simulink model "buck_soft_start_logic"  (R2024b)
settings: Solver=ode4  StartTime=0.0  StopTime=0.018  FixedStep=5e-7  RelTol=1e-3
undefined symbols (not defined in the file): DiscIntNeverNeededParam
libraries: simulink x1
settings Model: Creator=ww  LastModifiedBy=ww

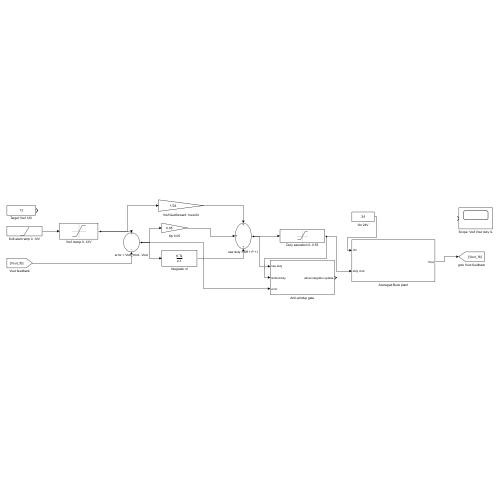
[thumbnail: Simulink's stored preview of the top-level diagram]
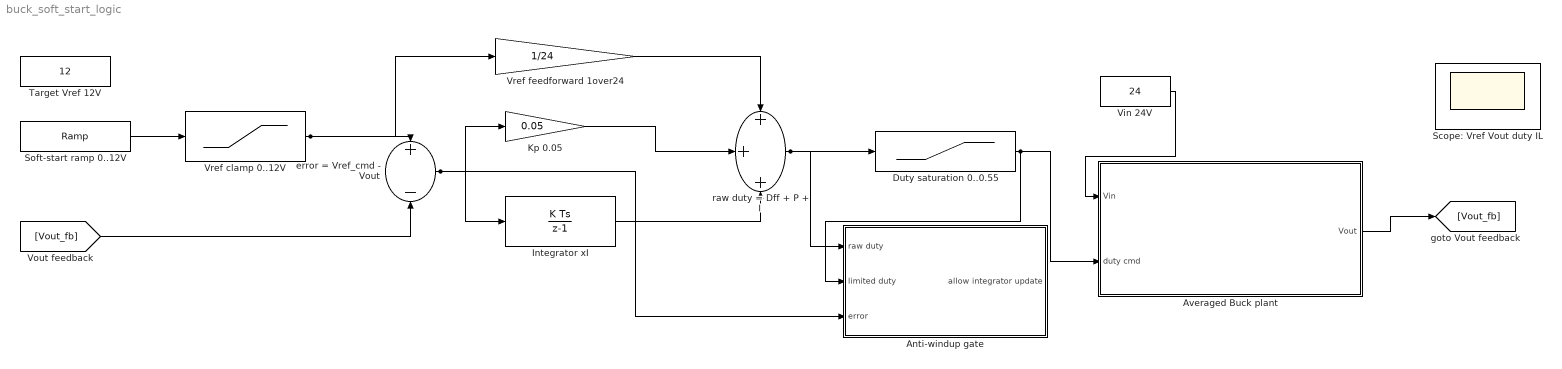
== system buck_soft_start_logic ==
  Anti-windup gate : Subsystem
  Averaged Buck plant : Subsystem
  Duty saturation 0..0.55 : Saturate  UpperLimit=0.55  LowerLimit=0
  Integrator xI : DiscreteIntegrator  gainval=200  SampleTime=5e-6  ICPrevOutput=DiscIntNeverNeededParam  ICPrevScaledInput=DiscIntNeverNeededParam
  Kp 0.05 : Gain  Gain=0.05
  Scope: Vref Vout duty IL : Scope
  Soft-start ramp 0..12V : simulink/Sources/Ramp  slope=12/0.005  start=0  InitialOutput=0
  Target Vref 12V : Constant  Value=12
  Vin 24V : Constant  Value=24
  Vref clamp 0..12V : Saturate  UpperLimit=12  LowerLimit=0
  Vref feedforward 1over24 : Gain  Gain=1/24
  error = Vref_cmd - Vout : Sum  Inputs=+-
  raw duty = Dff + P + I : Sum  Inputs=+++
  wires:
  Soft-start ramp 0..12V/1 -> Vref clamp 0..12V/1
  Vref clamp 0..12V/1 -> error = Vref_cmd - Vout/1, Vref feedforward 1over24/1
  [Vout_fb] -> error = Vref_cmd - Vout/2
  error = Vref_cmd - Vout/1 -> Kp 0.05/1, Integrator xI/1, Anti-windup gate/3(error)
  Vref feedforward 1over24/1 -> raw duty = Dff + P + I/1
  Kp 0.05/1 -> raw duty = Dff + P + I/2
  Integrator xI/1 -> raw duty = Dff + P + I/3
  raw duty = Dff + P + I/1 -> Duty saturation 0..0.55/1, Anti-windup gate/1(raw duty)
  Duty saturation 0..0.55/1 -> Anti-windup gate/2(limited duty), Averaged Buck plant/2(duty cmd)
  Vin 24V/1 -> Averaged Buck plant/1(Vin)
  Averaged Buck plant/1(Vout) -> [Vout_fb]

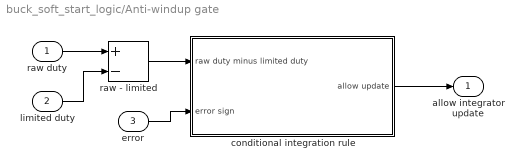
== system buck_soft_start_logic/Anti-windup gate ==
  raw duty : Inport
  limited duty : Inport  Port=2
  error : Inport  Port=3
  conditional integration rule : Subsystem
  raw - limited : Sum  Inputs=+-
  allow integrator update : Outport
  wires:
  error/1 -> conditional integration rule/2(error sign)
  raw - limited/1 -> conditional integration rule/1(raw duty minus limited duty)
  raw duty/1 -> raw - limited/1
  limited duty/1 -> raw - limited/2
  conditional integration rule/1(allow update) -> allow integrator update/1

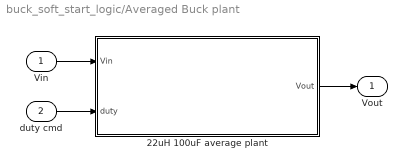
== system buck_soft_start_logic/Averaged Buck plant ==
  Vin : Inport
  duty cmd : Inport  Port=2
  22uH 100uF average plant : Subsystem
  Vout : Outport
  wires:
  Vin/1 -> 22uH 100uF average plant/1(Vin)
  duty cmd/1 -> 22uH 100uF average plant/2(duty)
  22uH 100uF average plant/1(Vout) -> Vout/1

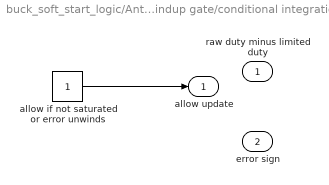
== system buck_soft_start_logic/Anti-windup gate/conditional integration rule ==
  raw duty minus limited duty : Inport
  error sign : Inport  Port=2
  allow if not saturated or error unwinds : Constant
  allow update : Outport
  wires:
  allow if not saturated or error unwinds/1 -> allow update/1

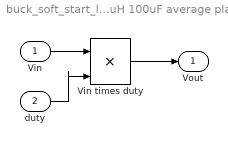
== system buck_soft_start_logic/Averaged Buck plant/22uH 100uF average plant ==
  Vin : Inport
  duty : Inport  Port=2
  Vin times duty : Product
  Vout : Outport
  wires:
  Vin times duty/1 -> Vout/1
  duty/1 -> Vin times duty/2
  Vin/1 -> Vin times duty/1
